simulink model "sfcndemo_sfun_udt"  (Simulink 7.6)
settings: Solver=ode1  StartTime=0.0  StopTime=10.0  FixedStep=0.05  RelTol=1e-3
Description:
  | User-defined data type in C-MEX S-function
settings Model: Creator=The MathWorks Inc.  ExtModeAutoUpdateStatusClock=off
settings SolverCC: ZeroCrossControl=DisableAll
settings DataIOCC: SaveOutput=off  SaveTime=off
settings OptimizationCC: BlockReduction=off  BooleanDataType=off  InitFltsAndDblsToZero=on
settings DebuggingCC: SaveWithParameterizedLinksMsg=none  SignalResolutionControl=TryResolveAllWithWarning  SolverPrmCheckMsg=none  MultiTaskDSMMsg=warning  MultiTaskCondExecSysMsg=none
settings HardwareCC: TargetUnknown=on
settings RTWCC: RetainRTWFile=on  IncludeERTFirstTime=on
settings CodeAppCC: CustomSymbolStrFcn=$F$N$M
settings GRTTargetCC: TargetFcnLib=ansi_tfl_tmw.mat

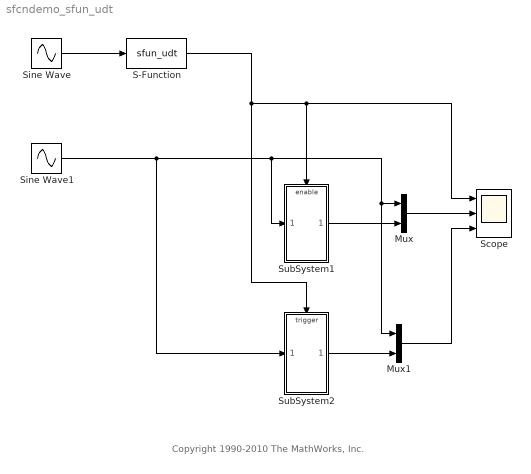
== system sfcndemo_sfun_udt ==
  note: Copyright 1990-2010 The MathWorks, Inc.
  Mux : Mux  Inputs=2
  Mux1 : Mux  Inputs=2
  S-Function : S-Function  FunctionName=sfun_udt  EnableBusSupport=off
  Scope : Scope  NumInputPorts=3
      settings: YMin=-5~-5~-5  YMax=5~5~5
  Sine Wave : Sin  Amplitude=4.5  Frequency=1.5  SampleTime=0.05
  Sine Wave1 : Sin  Amplitude=4  SampleTime=0.05
  SubSystem1 : Subsystem  TreatAsAtomicUnit=on
  SubSystem2 : Subsystem  TreatAsAtomicUnit=on
  wires:
  Sine Wave/1 -> S-Function/1
  S-Function/1 -> SubSystem2/Trigger, SubSystem1/Enable, Scope/1
  Sine Wave1/1 -> SubSystem2/1(In1), SubSystem1/1(In1), Mux/1, Mux1/1
  Mux/1 -> Scope/2
  SubSystem1/1(Out1) -> Mux/2
  SubSystem2/1(Out1) -> Mux1/2
  Mux1/1 -> Scope/3

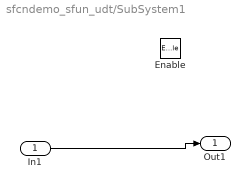
== system sfcndemo_sfun_udt/SubSystem1 ==
  In1 : Inport
  Enable : EnablePort
  Out1 : Outport
  wires:
  In1/1 -> Out1/1

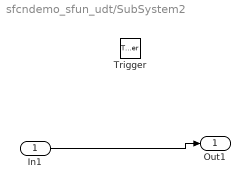
== system sfcndemo_sfun_udt/SubSystem2 ==
  In1 : Inport
  Trigger : TriggerPort
  Out1 : Outport
  wires:
  In1/1 -> Out1/1
